simulink model "chap7_1sim"  (Simulink 7.7)
settings: Solver=ode45  StartTime=0.0  StopTime=30  RelTol=1e-3
settings Model: Creator=ljk  LastModifiedBy=ljk  ExtModeTrigMode=oneshot  ExtModeArmWhenConnect=off
settings DataIOCC: LimitDataPoints=off  SignalLoggingName=sigsOut
settings OptimizationCC: BooleanDataType=off
settings DebuggingCC: SaveWithParameterizedLinksMsg=none  SignalResolutionControl=TryResolveAllWithWarning  SolverPrmCheckMsg=none  MultiTaskDSMMsg=warning  MultiTaskCondExecSysMsg=none  StrictBusMsg=None
settings HardwareCC: TargetUnknown=on
settings RTWCC: IncludeERTFirstTime=on

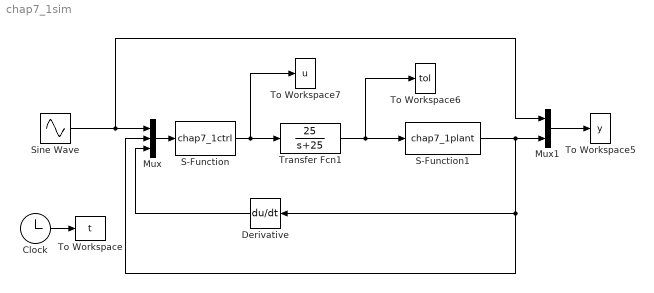
== system chap7_1sim ==
  Clock : Clock
  Derivative : Derivative
  Mux : Mux  Inputs=3
  Mux1 : Mux  Inputs=2
  S-Function : S-Function  FunctionName=chap7_1ctrl  EnableBusSupport=off
  S-Function1 : S-Function  FunctionName=chap7_1plant  EnableBusSupport=off
  Sine Wave : Sin  SampleTime=0
  To Workspace : ToWorkspace  VariableName=t  SampleTime=-1  SaveFormat=Array
  To Workspace5 : ToWorkspace  VariableName=y  SampleTime=-1  SaveFormat=Array
  To Workspace6 : ToWorkspace  VariableName=tol  SampleTime=-1  SaveFormat=Array
  To Workspace7 : ToWorkspace  VariableName=u  SampleTime=-1  SaveFormat=Array
  Transfer Fcn1 : TransferFcn  Numerator=[25]  Denominator=[1 25]
  wires:
  Mux/1 -> S-Function/1
  Derivative/1 -> Mux/3
  Sine Wave/1 -> Mux/1, Mux1/1
  Mux1/1 -> To Workspace5/1
  S-Function1/1 -> Derivative/1, Mux/2, Mux1/2
  S-Function/1 -> To Workspace7/1, Transfer Fcn1/1
  Clock/1 -> To Workspace/1
  Transfer Fcn1/1 -> S-Function1/1, To Workspace6/1
